simulink model "ModeloSyncGen4"  (R2014b)
settings: Solver=ode45  StartTime=0.0  StopTime=20  RelTol=1e-3
values from neighbouring files (symbols this model uses):
  delta0 = double(delta)    [CalcSteady1.m]    (also in Main2.m)
  J = (1/2)*(H*S)/(ws^2)    (= 7029.15711519)    [CalcSteady1.m]    (also in CalcSteady2.m; Main.m = 3.75; Main2.m = 18500)
  Lq = 5.61e-3    (= 0.00561)    [CalcSteady1.m]    (also in CalcSteady2.m; Main.m; Main2.m; SolverODE.m)
  phi_D0 = double(phi_d)    [CalcSteady1.m]    (also in Main2.m)
  phi_F0 = double(phi_f)    [CalcSteady1.m]    (also in Main2.m)
  phi_Q0 = double(phi_q)    [CalcSteady1.m]    (also in Main2.m)
  Rf = 0.985e-3    (= 0.000985)    [CalcSteady1.m]    (also in CalcSteady2.m; Main.m; Main2.m; SolverODE.m)
  Rs = 1.6e-3    (= 0.0016)    [CalcSteady1.m]    (also in CalcSteady2.m; Main.m; Main2.m; SolverODE.m)
  Tm0 = double(Tm)    [CalcSteady1.m]    (also in Main.m = Tm; Main2.m)
  Vf = Rf*If    [CalcSteady1.m]    (also in CalcSteady2.m; Main.m = double(Rf*If); Main2.m = double(Rf*If); SolverODE.m = Vf0)
  Vrms = 20e3    (= 20000)    [CalcSteady1.m]    (also in Main.m = 22000; Main2.m; SolverODE.m = 22000)
  Wm0 = double(ws)    [CalcSteady1.m]    (also in Main2.m)
settings Model: Creator=Eduardo Montilva  LastModifiedBy=Eduardo Montilva

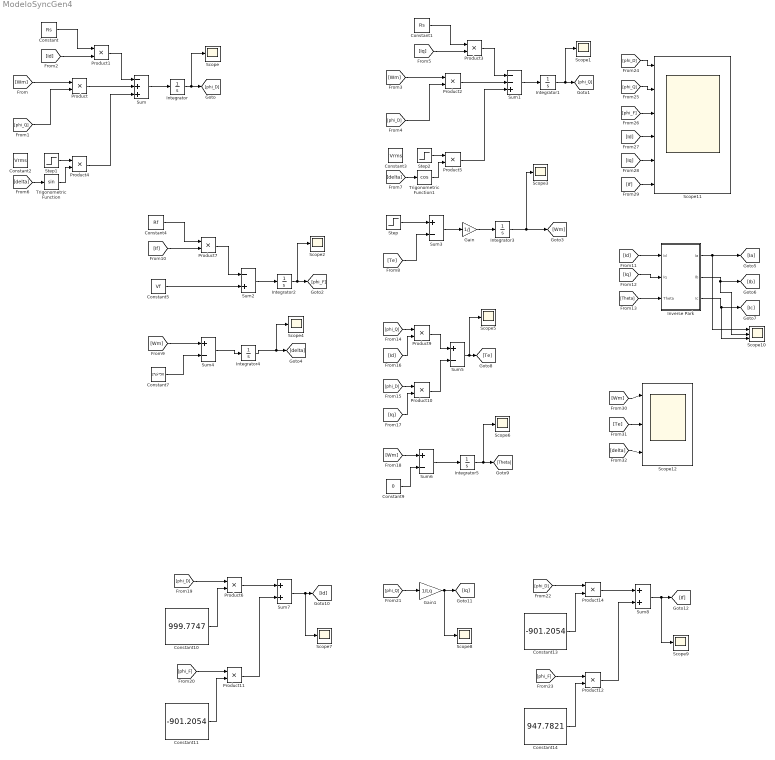
== system ModeloSyncGen4 ==
  Constant : Constant  Value=Rs
  Constant1 : Constant  Value=Rs
  Constant10 : Constant  Value=999.7747
  Constant11 : Constant  Value=-901.2054
  Constant13 : Constant  Value=-901.2054
  Constant14 : Constant  Value=947.7821
  Constant2 : Constant  Value=Vrms
  Constant3 : Constant  Value=Vrms
  Constant4 : Constant  Value=Rf
  Constant5 : Constant  Value=Vf
  Constant7 : Constant  Value=2*pi*50
  Constant9 : Constant  Value=0
  Gain : Gain  Gain=1/J
  Gain1 : Gain  Gain=1/Lq
  Integrator : Integrator  InitialCondition=phi_D0
  Integrator1 : Integrator  InitialCondition=phi_Q0
  Integrator2 : Integrator  InitialCondition=phi_F0
  Integrator3 : Integrator  InitialCondition=Wm0
  Integrator4 : Integrator  InitialCondition=delta0
  Integrator5 : Integrator
  Inverse Park : Subsystem
  Product{,1..7,9..12,14} (13 alike) : Product
  Scope{,1..9} (10 alike) : Scope
      Scope2 settings: SaveName=ScopeData2
      Scope3 settings: YMin=2100  YMax=3100  SaveName=ScopeData3
      Scope4 settings: SaveName=ScopeData4
      Scope5 settings: YMin=-4e+06  YMax=4e+06  SaveName=ScopeData5
      Scope6 settings: SaveName=ScopeData6
      Scope7 settings: SaveName=ScopeData7
      Scope8 settings: SaveName=ScopeData8
      Scope9 settings: SaveName=ScopeData9
  Scope10 : Scope  NumInputPorts=3
      settings: YMin=-5~-5~-5  YMax=5~5~5  SaveName=ScopeData10
  Scope11 : Scope  NumInputPorts=6
      settings: YMin=-5~-5~-5~-5~-5~-5  YMax=5~5~5~5~5~5  SaveName=ScopeData11
  Scope12 : Scope  NumInputPorts=3
      settings: YMin=-5~-5~-5  YMax=5~5~5  SaveName=ScopeData12
  Step : Step  Before=Tm0  After=Tm0  SampleTime=0
  Step1 : Step  Before=22e3  After=0  SampleTime=0
  Step2 : Step  Before=22e3  After=0  SampleTime=0
  Sum : Sum  Inputs=-++
  Sum1 : Sum  Inputs=--+
  Sum2 : Sum  Inputs=-+
  Sum{3..6} (4 alike) : Sum  Inputs=+-
  Sum7 : Sum
  Sum8 : Sum
  Trigonometric Function : Trigonometry
  Trigonometric Function1 : Trigonometry  Operator=cos
  wires:
  [Wm] -> Product/1
  [phi_Q] -> Product/2
  Product/1 -> Sum/2
  [Id] -> Product1/2
  Constant/1 -> Product1/1
  Product1/1 -> Sum/1
  Sum/1 -> Integrator/1
  Integrator/1 -> Scope/1, [phi_D]
  [Wm] -> Product2/1
  Product2/1 -> Sum1/2
  [Iq] -> Product3/2
  Constant1/1 -> Product3/1
  Product3/1 -> Sum1/1
  Sum1/1 -> Integrator1/1
  Integrator1/1 -> Scope1/1, [phi_Q]
  [phi_D] -> Product2/2
  [delta] -> Trigonometric Function/1
  Trigonometric Function/1 -> Product4/2
  [delta] -> Trigonometric Function1/1
  Trigonometric Function1/1 -> Product5/2
  [If] -> Product7/2
  Constant4/1 -> Product7/1
  Product7/1 -> Sum2/1
  Sum2/1 -> Integrator2/1
  Integrator2/1 -> Scope2/1, [phi_F]
  Constant5/1 -> Sum2/2
  Step/1 -> Sum3/1
  [Te] -> Sum3/2
  Sum3/1 -> Gain/1
  [Wm] -> Sum4/1
  Constant7/1 -> Sum4/2
  Sum4/1 -> Integrator4/1
  Integrator4/1 -> Scope4/1, [delta]
  [phi_Q] -> Product9/1
  [phi_D] -> Product10/1
  [Iq] -> Product10/2
  [Id] -> Product9/2
  Product10/1 -> Sum5/2
  Product9/1 -> Sum5/1
  Sum5/1 -> Scope5/1, [Te]
  [Wm] -> Sum6/1
  Constant9/1 -> Sum6/2
  Sum6/1 -> Integrator5/1
  Integrator5/1 -> Scope6/1, [Theta]
  [phi_D] -> Product6/1
  Constant10/1 -> Product6/2
  Product6/1 -> Sum7/1
  Constant11/1 -> Product11/2
  [phi_F] -> Product11/1
  Product11/1 -> Sum7/2
  [phi_D] -> Product14/1
  Constant13/1 -> Product14/2
  Product14/1 -> Sum8/1
  Constant14/1 -> Product12/2
  [phi_F] -> Product12/1
  Product12/1 -> Sum8/2
  Sum8/1 -> Scope9/1, [If]
  Sum7/1 -> Scope7/1, [Id]
  Gain/1 -> Integrator3/1
  Integrator3/1 -> [Wm], Scope3/1
  Product4/1 -> Sum/3
  Product5/1 -> Sum1/3
  [Id] -> Inverse Park/1(Id)
  [Iq] -> Inverse Park/2("Iq ")
  [Theta] -> Inverse Park/3(Theta)
  Inverse Park/1(Ia) -> Scope10/1, [Ia]
  Inverse Park/2(Ib) -> Scope10/2, [Ib]
  Inverse Park/3(Ic) -> Scope10/3, [Ic]
  [phi_Q] -> Gain1/1
  Gain1/1 -> Scope8/1, [Iq]
  [phi_D] -> Scope11/1
  [phi_Q] -> Scope11/2
  [phi_F] -> Scope11/3
  [Id] -> Scope11/4
  [Iq] -> Scope11/5
  [If] -> Scope11/6
  [Wm] -> Scope12/1
  [Te] -> Scope12/2
  [delta] -> Scope12/3
  Step1/1 -> Product4/1
  Step2/1 -> Product5/1

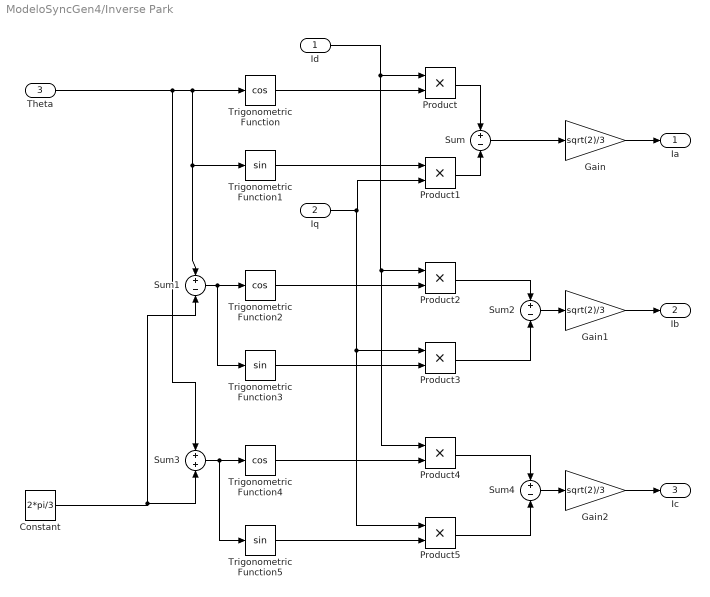
== system ModeloSyncGen4/Inverse Park ==
  Id : Inport
  "Iq " : Inport  Port=2
  Theta : Inport  Port=3
  Constant : Constant  Value=2*pi/3
  Gain : Gain  Gain=sqrt(2)/3
  Gain1 : Gain  Gain=sqrt(2)/3
  Gain2 : Gain  Gain=sqrt(2)/3
  Product{,1..5} (6 alike) : Product
  Sum{,1..2,4} (4 alike) : Sum  Inputs=+-
  Sum3 : Sum
  Trigonometric Function : Trigonometry  Operator=cos
  Trigonometric Function1 : Trigonometry
  Trigonometric Function2 : Trigonometry  Operator=cos
  Trigonometric Function3 : Trigonometry
  Trigonometric Function4 : Trigonometry  Operator=cos
  Trigonometric Function5 : Trigonometry
  Ia : Outport
  Ib : Outport  Port=2
  Ic : Outport  Port=3
  wires:
  Gain2/1 -> Ic/1
  Product2/1 -> Sum2/1
  Product3/1 -> Sum2/2
  Sum3/1 -> Trigonometric Function5/1, Trigonometric Function4/1
  Id/1 -> Product/1, Product4/1, Product2/1
  Trigonometric Function4/1 -> Product4/2
  Gain1/1 -> Ib/1
  Sum1/1 -> Trigonometric Function3/1, Trigonometric Function2/1
  Constant/1 -> Sum1/2, Sum3/2
  Sum2/1 -> Gain1/1
  Trigonometric Function2/1 -> Product2/2
  Product/1 -> Sum/1
  Trigonometric Function/1 -> Product/2
  "Iq "/1 -> Product5/1, Product3/1, Product1/2
  Gain/1 -> Ia/1
  Trigonometric Function1/1 -> Product1/1
  Product1/1 -> Sum/2
  Sum/1 -> Gain/1
  Product5/1 -> Sum4/2
  Trigonometric Function5/1 -> Product5/2
  Product4/1 -> Sum4/1
  Sum4/1 -> Gain2/1
  Trigonometric Function3/1 -> Product3/2
  Theta/1 -> Sum3/1, Trigonometric Function1/1, Sum1/1, Trigonometric Function/1
